simulink model "cam_model"  (R2024b)
settings: Solver=FixedStepDiscrete  StartTime=0.0  StopTime=10  FixedStep=0.001  MaxStep=0.005  RelTol=1e-3
values from neighbouring files (symbols this model uses):
  del_theta = beam_defl    [sim_setup.m]    (also in sim_setup_1.m)
  del_theta0 = const.init_deflection    [sim_setup.m]    (also in sim_setup_1.m)
  diff_del = diff(del_theta)/dTheta    [sim_setup.m]    (also in sim_setup_1.m)
  J = 0.0001    [sim_setup.m]    (also in sim_setup_1.m = 9.466956e-05)
  k = const.beam_stiffness    [sim_setup.m]    (also in sim_setup_1.m)
  T_ang = ang(1:length(ang)-1)    [sim_setup.m]    (also in sim_setup_1.m)
undefined symbols (not defined in the file or in its folder): ang, DiscIntNeverNeededParam
libraries: simulink_extras x1
settings Model: Creator=HNGG  LastModifiedBy=divg2
settings OptimizationCC: ReuseModelBlockBuffer=off
settings RTWCC: GPUComputeCapability=3.5

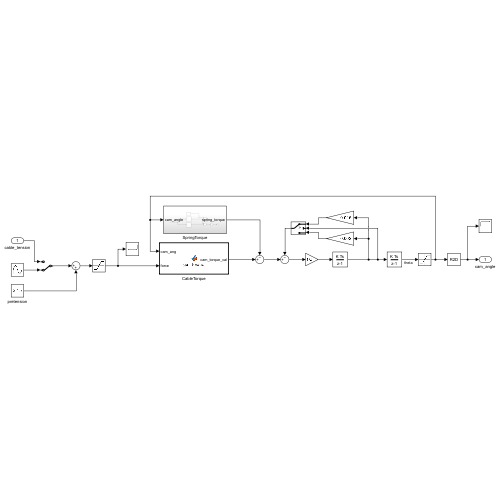
[thumbnail: Simulink's stored preview of the top-level diagram]
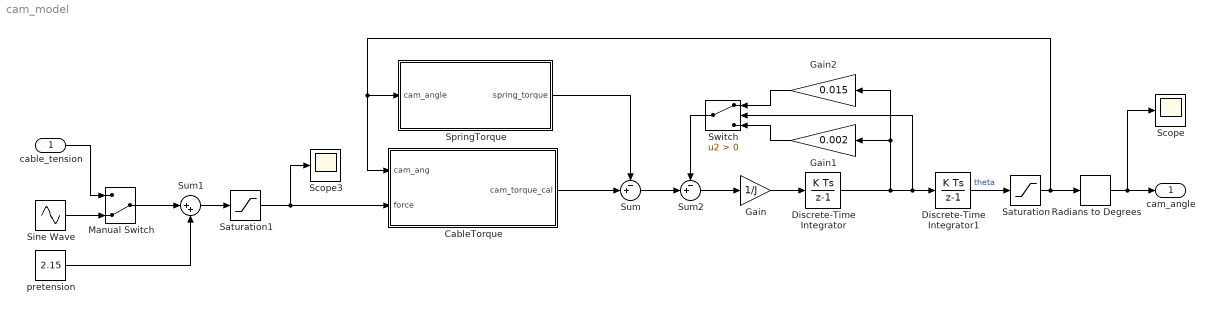
== system cam_model ==
  cable_tension : Inport
  CableTorque : MATLAB Function  TreatAsAtomicUnit=on
  Discrete-Time Integrator : DiscreteIntegrator  SampleTime=-1  ICPrevOutput=DiscIntNeverNeededParam  ICPrevScaledInput=DiscIntNeverNeededParam
  Discrete-Time Integrator1 : DiscreteIntegrator  SampleTime=-1  ICPrevOutput=DiscIntNeverNeededParam  ICPrevScaledInput=DiscIntNeverNeededParam
  Gain : Gain  Gain=1/J
  Gain1 : Gain  Gain=0.002
  Gain2 : Gain  Gain=0.015
  Manual Switch : ManualSwitch  CurrentSetting=0
  Radians to Degrees : simulink_extras/Transformations/Radians to Degrees
  Saturation : Saturate  UpperLimit=70 * pi/180  LowerLimit=0
  Saturation1 : Saturate  UpperLimit=8  LowerLimit=2.15
  Scope : Scope
  Scope3 : Scope
  Sine Wave : Sin  Frequency=5*pi  SampleTime=0
  SpringTorque : Subsystem
  Sum : Sum  Inputs=-+|
  Sum1 : Sum  Inputs=|++
  Sum2 : Sum  Inputs=-+|
  Switch : Switch  Criteria=u2 > Threshold  SaturateOnIntegerOverflow=off  InputSameDT=off
  pretension : Constant  Value=2.15
  cam_angle : Outport
  wires:
  Discrete-Time Integrator/1 -> Gain1/1, Gain2/1, Switch/2, Discrete-Time Integrator1/1
  Gain/1 -> Discrete-Time Integrator/1
  Sum/1 -> Sum2/2
  CableTorque/1(cam_torque_cal) -> Sum/2
  Sum2/1 -> Gain/1
  SpringTorque/1(spring_torque) -> Sum/1
  Radians to Degrees/1 -> Scope/1, cam_angle/1
  pretension/1 -> Sum1/2
  Sum1/1 -> Saturation1/1
  cable_tension/1 -> Manual Switch/1
  Manual Switch/1 -> Sum1/1
  Saturation/1 -> SpringTorque/1(cam_angle), CableTorque/1(cam_ang), Radians to Degrees/1
  Discrete-Time Integrator1/1 -> Saturation/1  "theta"
  Sine Wave/1 -> Manual Switch/2
  Saturation1/1 -> Scope3/1, CableTorque/2(force)
  Switch/1 -> Sum2/1
  Gain2/1 -> Switch/1
  Gain1/1 -> Switch/3

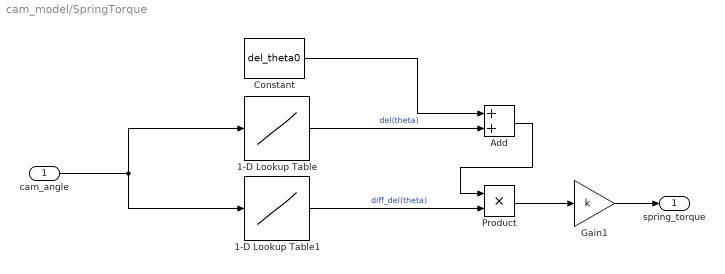
== system cam_model/SpringTorque ==
  cam_angle : Inport
  1-D Lookup Table : Lookup_n-D  NumberOfTableDimensions=1  BreakpointsForDimension1=ang  Table=del_theta  InternalRulePriority=Speed  RndMeth=Simplest
  1-D Lookup Table1 : Lookup_n-D  NumberOfTableDimensions=1  BreakpointsForDimension1=T_ang  Table=diff_del  InternalRulePriority=Speed  RndMeth=Simplest
  Add : Sum
  Constant : Constant  Value=del_theta0
  Gain1 : Gain  Gain=k
  Product : Product
  spring_torque : Outport
  wires:
  cam_angle/1 -> 1-D Lookup Table1/1, 1-D Lookup Table/1
  1-D Lookup Table1/1 -> Product/2  "diff_del(theta)"
  Gain1/1 -> spring_torque/1
  Constant/1 -> Add/1
  Add/1 -> Product/1
  Product/1 -> Gain1/1
  1-D Lookup Table/1 -> Add/2  "del(theta)"

== matlab function cam_model/CableTorque ==
  data: cam_ang input; cam_torque_cal output; force input
function cam_torque_cal = get_torque(cam_ang,force)
r = 5/1000;
l_p3 = 55/1000;
P1 = [-23.61/1000; 18/1000; 0];
P2 = [-36.04/1000; 61.25/1000; 0];
theta = deg2rad(59)+cam_ang;


P3 = [l_p3*cos(theta); l_p3*sin(theta); 0];
d_13 = P1-P3;
d_23 = P2-P3;

beta1 = asin(2*r/norm(d_13));
beta2 = asin(2*r/norm(d_23));


% for P1
a1 = [0;-1;0]; b1 = -d_13;
psi1 = acos(dot(a1,b1)/norm(a1)/norm(b1));
c1 = cross(a1,b1);
if c1(3)<0
    psi1 = 2*pi - psi1;
end

phi1 = -beta1+psi1;
r1 = r*[cos(phi1);sin(phi1);0];

a2 = -d_23; b2 = [0;1;0];
psi2 = acos(dot(a2,b2)/norm(a2)/norm(b2));
c2 = cross(a2,b2);
if c2(3)<0
    psi2 = 2*pi - psi2;
end

phi2 = beta2-psi2;
r2 = r*[cos(phi2);sin(phi2);0];

y1 = d_13 + 2*r1;
tau1 = force*cross(P3-r1,y1/norm(y1));
y2 = d_23 + 2*r2;
tau2 = force*cross(P3-r2,y2/norm(y2));

tau = tau1+tau2;
cam_torque_cal = tau(3);

end
